simulink model "flightControlSystem"  (R2025b)
settings: Solver=ode3  StartTime=0  StopTime=TFinal  FixedStep=Ts  RelTol=1e-3  EnableMultiTasking=on
undefined symbols (not defined in the file): codertarget, Controller, DiscIntNeverNeededParam, Discrete, Estimator, g, init, orient_ref, pos_ref, Sensors, Time, Ts, var_acc_angle_N, var_bias_gyr_N, var_gyro_p_N, Vehicle
libraries: simulink x37, matrix_library x15, slpidlib x4, ctrlSharedLib x4, sharedtransform x3, visiontextngfix x3, simulink_extras x2, parrotlib x2, visionsinks x2
(part 3 of 4)

== system flightControlSystem/Control System/State Estimator/XY Position Estimator/EstimatorVelocity/xy velocity w//o angular velocity compensation ==
  note: Optical flow raw readings are converted to velocity in m/s based on the estimated altitude
  optical_flow : Inport
  z_estimate : Inport  Port=2
  " " : Product  Inputs=**
  Compare To Constant : simulink/Logic and Bit Operations/Compare To Constant  relop=<  const=200*4  OutDataTypeStr=boolean
  Counter Free-Running : simulink/Sources/Counter Free-Running  NumBits=32  tsamp=-1
  Gain : Gain  Gain=-1
  Select dxy : Selector  InputPortWidth=3  IndexOptions=Index vector (dialog)  Indices=[1 2]  OutputSizes=1
  Switch : Switch  Criteria=u2 > Threshold  SaturateOnIntegerOverflow=off  InputSameDT=off
  opticalFlowErrorCorrect : Gain  Gain=1.15
  optical_flow_dx_dy : Outport
  wires:
  Select dxy/1 -> optical_flow_dx_dy/1  "optical_flow_dx_dy"
  " "/1 -> opticalFlowErrorCorrect/1
  opticalFlowErrorCorrect/1 -> Switch/3
  Gain/1 -> " "/2
  Switch/1 -> Select dxy/1
  Counter Free-Running/1 -> Compare To Constant/1
  Compare To Constant/1 -> Switch/2
  optical_flow/1 -> " "/1, Switch/1
  z_estimate/1 -> Gain/1

== matlab function flightControlSystem/Image Processing System/MATLAB Function ==
  data: r input; rgb output; g input; b input
function rgb = fcn(r,g,b)

rgb = cat(3,r,g,b);

end

== matlab function flightControlSystem/Control System/Controller/Position Controller/Position error transformation (Earth to Body frame) ==
  data: yaw input; xy_err_earth input; xy_err_body output
function xy_err_body = fcn(yaw,xy_err_earth)

transformation = [cos(yaw), sin(yaw); -sin(yaw),  cos(yaw)];
xy_err_body = transformation * xy_err_earth;


end

== stateflow chart flightControlSystem/Control System/Path Planning/Chart ==
  state Move6
    entry:
    X_out = X_a;
    Y_out = Y_a;
    Z_out = Z_a;
    T = 0;
    X_b_dot_max = 0.25 / (0.005*0.7);
    Y_b_dot_max = 0.1 / (0.005*0.7);
    %Y_b_dot_max = (0.1 * kp_xb) / (0.005*0.7);
    during:
    T = (T + Del_T);
    X_b_dot = (kp_xb) * X_b_dot_max * min(0.2*T,1);
    Y_b_dot  = -y_kp * Y_b_dot_max * min(T,1);
    X_out = X_a + ( X_b_dot * cos(Yaw_out*(pi/180) ) + Y_b_dot * sin(Yaw_out*(pi/180)) )*Del_T;
    Y_out = Y_a + ( - X_b_dot * sin(Yaw_out*(pi/180) ) + Y_b_dot * cos(Yaw_out*(pi/180)) )*Del_T;
  state Forward_case
    entry:
    T = 0;
    X_out = X_a;
    Y_out = Y_a;
    Z_out = Z_a;
    X_b_dot_max = 0.05 / (0.005*0.7); % 0.1 before, with oscillations
    Y_b_dot_max = 0.05 / (0.005*0.7);
    during:
    T = (T + Del_T);
    X_b_dot = (kp_xb) * X_b_dot_max * min(0.2*T,1);
    Y_b_dot  = -y_kp * Y_b_dot_max * min(T,1);
    X_out = X_a + ( X_b_dot * cos(Yaw_out*(pi/180) ) + Y_b_dot * sin(Yaw_out*(pi/180)) )*Del_T;
    Y_out = Y_a + ( - X_b_dot * sin(Yaw_out*(pi/180) ) + Y_b_dot * cos(Yaw_out*(pi/180)) )*Del_T;
    Yaw_out = Yaw_a +  10 * Yaw_kp * min(0.5*T,1);
  state Right_move
    entry:
    T = 0;
    X_out = X_a;
    Y_out = Y_a;
    Z_out = Z_a;
    X_b_dot_max = 0.05 / (0.005*0.7); % 0.1 before, with oscillations
    Y_b_dot_max = 0.25 / (0.005*0.7);
    during:
    T = (T + Del_T);
    X_b_dot = x_kp * X_b_dot_max * min(T,1);
    Y_b_dot  = kp_yb_r * Y_b_dot_max * min(0.5*T,1);
    X_out = X_a + ( X_b_dot * cos(Yaw_out*(pi/180) ) + Y_b_dot * sin(Yaw_out*(pi/180)) )*Del_T;
    Y_out = Y_a + ( - X_b_dot * sin(Yaw_out*(pi/180) ) + Y_b_dot * cos(Yaw_out*(pi/180)) )*Del_T;
    %Yaw_out = Yaw_a - 2 * yaw_kp_turn_right * min(T,1);
  state Right_pre_move
    entry:
    T = 0;
    X_out = X_a;
    Y_out = Y_a;
    Z_out = Z_a;
    X_b_dot_max = 0.05 / (0.005*0.7); % 0.1 before, with oscillations
    Y_b_dot_max = 0.05 / (0.005*0.7);
    during:
    T = (T + Del_T);
    X_b_dot =  x_kp * X_b_dot_max * min(T,1);
    Y_b_dot  = kp_yb_r * Y_b_dot_max * min(0.5*T, 1);
    X_out = X_a + ( X_b_dot * cos(Yaw_out*(pi/180) ) + Y_b_dot * sin(Yaw_out*(pi/180)) )*Del_T;
    Y_out = Y_a + ( - X_b_dot * sin(Yaw_out*(pi/180) ) + Y_b_dot * cos(Yaw_out*(pi/180)) )*Del_T;
    Yaw_out = Yaw_a - 10 * yaw_kp_turn_right * min(0.5*T,1);
  state takeoff1
    entry:
    X_out = X_a;
    Y_out = Y_a;
    Z_out = Z_a;
    Yaw_out = Yaw_a;
    during:
    Z_out = -1.1;
  state Initial_Yaw1
    entry:
    T = 0;
    X_out = X_a;
    Y_out = Y_a;
    Z_out = Z_a;
    Yaw_out = Yaw_a;
    during:
    T = (T + Del_T);
    Yaw_out = Yaw_a + 5 * Yaw_kp * min(0.5*T, 1) * n;
  state Move1
    entry:
    T = 0;
    X_b_dot_max = 0.25 / (0.005*0.7);
    Y_b_dot_max = 0.1 / (0.005*0.7);
    %Y_b_dot_max = (0.15 * kp_xb) / (0.005*0.7);
    Yaw_out = Yaw_a;
    during:
    T = (T + Del_T);
    X_b_dot = kp_xb * X_b_dot_max * min(0.2 *T,1);
    Y_b_dot  = -y_kp * Y_b_dot_max * min(T,1);
    X_out = X_a + ( X_b_dot * cos(Yaw_out*(pi/180) ) + Y_b_dot * sin(Yaw_out*(pi/180)) )*Del_T;
    Y_out = Y_a + ( - X_b_dot * sin(Yaw_out*(pi/180) ) + Y_b_dot * cos(Yaw_out*(pi/180)) )*Del_T;
  state Pre_land [commented out]
    entry:
    X_out = X_a;
    Y_out = Y_a;
    Z_out = Z_a;
    Yaw_out = Yaw_a;
    during:
    X_out = X_a;
    Y_out = Y_a;
    Z_out = Z_a;
    Yaw_out = Yaw_a;
  state Pre_land2 [commented out]
    entry:
    X_out = X_a;
    Y_out = Y_a;
    Z_out = Z_a;
    Yaw_out = Yaw_a;
    during:
    X_out = X_a;
    Y_out = Y_a;
    Z_out = Z_a;
  state Left_pre_move
    entry:
    T = 0;
    X_out = X_a;
    Y_out = Y_a;
    Z_out = Z_a;
    X_b_dot_max = 0.05 / (0.005*0.7); % 0.1 before, with oscillations
    Y_b_dot_max = -0.05 / (0.005*0.7);
    during:
    T = (T + Del_T);
    X_b_dot =  x_kp * X_b_dot_max * min(T,1);
    Y_b_dot  = kp_yb_l * Y_b_dot_max * min(0.5*T, 1);
    X_out = X_a + ( X_b_dot * cos(Yaw_out*(pi/180) ) + Y_b_dot * sin(Yaw_out*(pi/180)) )*Del_T;
    Y_out = Y_a + ( - X_b_dot * sin(Yaw_out*(pi/180) ) + Y_b_dot * cos(Yaw_out*(pi/180)) )*Del_T;
    Yaw_out = Yaw_a - 10 * yaw_kp_turn_left * min(0.5*T, 1);
  state Try_yaw
    entry:
    T = 0;
    X_out = X_a;
    Y_out = Y_a;
    Z_out = Z_a;
    Yaw_out = Yaw_a;
    during:
    T = (T + Del_T);
    Yaw_out = Yaw_a + 2 * n * yaw_dir_fs * min(0.5*T,1);
    %Yaw_out = Yaw_a + 2*n*min(T,1);
  state Left_move
    entry:
    T = 0;
    X_out = X_a;
    Y_out = Y_a;
    Z_out = Z_a;
    X_b_dot_max = 0.05 / (0.005*0.7); % 0.1 before, with oscillations
    Y_b_dot_max = -0.25 / (0.005*0.7);
    during:
    T = (T + Del_T);
    X_b_dot = x_kp * X_b_dot_max * min(T,1);
    Y_b_dot  = kp_yb_l * Y_b_dot_max * min(0.5*T,1);
    X_out = X_a + ( X_b_dot * cos(Yaw_out*(pi/180) ) + Y_b_dot * sin(Yaw_out*(pi/180)) )*Del_T;
    Y_out = Y_a + ( - X_b_dot * sin(Yaw_out*(pi/180) ) + Y_b_dot * cos(Yaw_out*(pi/180)) )*Del_T;
  state Pre_land1 [commented out]
    entry:
    X_out = X_a;
    Y_out = Y_a;
    Z_out = Z_a;
    Yaw_out = Yaw_a;
    during:
    X_out = X_a;
    Y_out = Y_a;
    Z_out = Z_a;
  Move6 -> Move1 [order 1] : [kp_xb <= 0.05 && valid_u == 0]
  Forward_case -> Move6 [order 1] : [abs(yaw_kp_2) <= 0.02 && kp_xb >= 0.95 && kp_xb_l >= 0.95 && kp_xb_r >= 0.95]
  Move6 -> Forward_case [order 2] : [kp_xb <= 0.05]
  Move1 -> Forward_case [order 1] : [abs(yaw_kp_2) >= 0.1 && valid_u == 1 && kp_xb <= 0.05 ]
  Forward_case -> Move1 [order 2] : [kp_xb <= 0.05 && valid_u == 0]
  takeoff1 -> Move1 [order 1] : after(3,sec) [Yaw_kp == 0 && kp_xb >= 0.9]
  Right_move -> Move1 [order 2] : [kp_yb_r <= 0.05 && valid_r == 0 && (valid_l ==1 || valid_u == 1)]
  Move1 -> Right_pre_move [order 2] : [valid_u == 0 && valid_r == 1 && kp_xb <= 0.02]
  Right_pre_move -> Right_move [order 1] : [kp_yb_r >= 0.95 && abs(yaw_kp_turn_right) <= 0.02 && valid_r == 1]
  (default) -> takeoff1
  takeoff1 -> Initial_Yaw1 [order 2] : after(3,sec) [Yaw_kp ~= 0 ]{n = 1}
  Initial_Yaw1 -> Move1 : [Yaw_kp == 0 && kp_xb >= 0.95 && kp_xb_l >= 0.95 && kp_xb_r >= 0.95]{n = 1}
  Move1 -> Initial_Yaw1 [commented out] : [valid_u == 0 && valid_l == 0 && valid_r == 0]
  Right_pre_move -> Move1 [order 2] : [kp_yb_r <= 0.05 && valid_r == 0]
  Move1 -> Try_yaw [order 4] : [valid_u == 0 && valid_l == 0 && valid_r == 0 && land_flag == 0]
  Right_move -> Right_pre_move [order 3] : [kp_yb_r <= 0.5 && valid_r == 1 && abs(yaw_kp_turn_right) >= 0.05]
  Try_yaw -> Move1 : [valid_u == 1]
  Move1 -> Pre_land [commented out] : [land_flag == 1 && (valid_l == 0 || valid_r == 0)]
  Left_move -> Move1 [order 2] : [kp_yb_l <= 0.05 && valid_l == 0 && ( valid_r == 1 || valid_u == 1) ]
  Left_pre_move -> Move1 [order 1] : [kp_yb_l <= 0.05 && valid_l == 0]
  Move1 -> Left_pre_move [order 3] : [valid_u == 0 && valid_l == 1 && kp_xb <= 0.02]
  Right_move -> Try_yaw [order 1] : [kp_yb_r <= 0.05 && valid_r == 0]{n = -1}
  Right_move -> Pre_land2 [commented out] : [land_flag == 1 && (valid_l == 0 || valid_r == 0)]
  Left_move -> Left_pre_move [order 3] : [kp_yb_l <= 0.5 && valid_l == 1 && abs(yaw_kp_turn_left) >= 0.05]
  Left_pre_move -> Left_move [order 2] : [kp_yb_l >= 0.95 && abs(yaw_kp_turn_left) <= 0.02 && valid_l == 1]
  Left_move -> Try_yaw [order 1] : [kp_yb_l <= 0.05 && valid_l == 0]{n = 1}
  Try_yaw -> Pre_land1 [commented out] : [land_flag == 1 && (valid_l == 0 || valid_r == 0)]
  data: y_kp input; Yaw_kp input; kp_xb input; yaw_kp_turn_right input; valid_r input; kp_yb_r input; yaw_kp_down input; yaw_kp_turn_left input; valid_d input; valid_l input; valid_u input; yaw_kp_2 input; kp_yb_l input; error_yaw input; kp_xb_l input; kp_xb_r input; x_kp input; land_flag input; land_dir input; yaw_dir_fs input; Del_T input; X_a input; Y_a input; Z_a input; Yaw_a input; X_out output; Y_out output; Z_out output; Yaw_out output; X_b_dot local; Y_b_dot local; T local; X_b_dot_max local; Y_b_dot_max local; a local; n local

== matlab function flightControlSystem/Image Processing System/Yaw_gain_finder ==
  data: u input; control output; L_sum input; R_sum input; valid_u output; temp output; error_yaw output
function [control, valid_u, temp, error_yaw] = processVector(u, L_sum, R_sum)

N = 160;
center = 80;
deadband = 2;

max_error = center - 1 - deadband;  % adjust for deadband



first_idx = 0;
last_idx = 0;

best_first = 0;
best_last = 0;
best_dist = inf;

in_block = 0;

for i = 1:N
    
    if u(i) ~= 0
        
        if in_block == 0
            first_idx = i;
            in_block = 1;
        end
        
        last_idx = i;
        
    else
        
        if in_block == 1
            
            mid = (first_idx + last_idx)/2;
            dist = abs(mid - center);
            
            if dist < best_dist
                best_dist = dist;
                best_first = first_idx;
                best_last = last_idx;
            end
            
            in_block = 0;
        end
        
    end
    
end

% Handle case if vector ended while still inside block
if in_block == 1
    mid = (first_idx + last_idx)/2;
    dist = abs(mid - center);
    
    if dist < best_dist
        best_first = first_idx;
        best_last = last_idx;
    end
end

first_idx = best_first;
last_idx  = best_last;

% ---- No detection ----
if first_idx == 0
    T_sum = L_sum + R_sum;
    dir_no_line = sign(T_sum);
    % if dir_no_line == 0
    %     dir_no_line = -1;
    % end
    control = dir_no_line * 2;   % search behaviour
    temp = 0;
    valid_u = 0;
    error_yaw = 1;
    return;
end



valid_u = 1;

% Middle of cluster
mid_index = (first_idx + last_idx)/2;
error = mid_index - center;


diff = (last_idx - first_idx);

first_diff = (mid_index-first_idx)/diff;
last_diff = (last_idx-mid_index)/diff;

if first_diff == 0.5 && last_diff ==0.5
    error_yaw =0;
else
    error_yaw = 1;
end

% ---- Deadband ----
if abs(error) <= deadband
    control = 0;
    temp = control;
    error_yaw = 0;
    return;
end

% Remove deadband offset
if error > 0
    error = error - deadband;
else
    error = error + deadband;
end

% Normalize
norm_error = (error / max_error) * 2;

% % ---- Quadratic shaping ----

control = -sign(norm_error) * (abs(norm_error))^2;
% control = - (0.7 * norm_error + 0.3 * norm_error * abs(norm_error));
temp = control;

%
% gain = 2.5;  % tune 1 to 4
% control = -tanh(gain * norm_error);
% temp = control;

== matlab function flightControlSystem/Image Processing System/Forward_gain ==
  data: forward_vector input; kp_forward output
function kp_forward  = fcn(forward_vector)

first_idx = 0;
last_idx  = 0;

% Scan vector manually
for i = 1:50
    if forward_vector(i) ~= 0
        if first_idx == 0
            first_idx = i;
        end
        last_idx = i;
    end
end

s = last_idx - first_idx;
kp_forward = s/50;

end

== matlab function flightControlSystem/Image Processing System/MATLAB Function1 ==
  data: binary_img input; theta_to_go output
function theta_to_go = findLineAngleFromCenter(binary_img)

rows = 120;
cols = 160;

center_r = 60;
center_c = 80;

sum_x = 0;
sum_y = 0;
count = 0;
angle_array = zeros(1000);

for r = 1:rows
    for c = 1:cols
        
        if binary_img(r,c) ~= 0
            
            % Vector from center to pixel
            x = -(c - center_c);
            y = -(center_r - r);   
            count = count + 1;
            theta = atan2d(y,x);
            theta = round(theta,2);
            angle_array(count)= theta;
        end
    end
end
% angle_array = round(angle_array, 1);
theta_to_go = mode(angle_array);


end

== matlab function flightControlSystem/Image Processing System/MATLAB Function2 ==
  data: Right_vector input; control output; valid_r output
function [control, valid_r] = fcn(Right_vector)

N = 105;
center = 45;
deadband = 1;

max_error = center - 1 - deadband;  % adjust for deadband

first_idx = 0;
last_idx  = 0;
in_block = 0;

% % Scan vector manually
% for i = 1:N
%     if Right_vector(i) ~= 0
%         if first_idx == 0
%             first_idx = i;
%         end
% 
%         last_idx = i;
%     end
% 
% end

for i = 1:N
    
    if Right_vector(i) ~= 0
        
        if in_block == 0
            first_idx = i;   % start of first block
            in_block = 1;
        end
        
        last_idx = i;        % update while inside block
        
    else
        % If we were inside a block and hit zero → block ended
        if in_block == 1
            break;           % STOP scanning
        end
    end
    
end



% ---- No detection ----
if first_idx == 0
    control = 0;   % search behaviour
    valid_r = 0;
    return;
end

valid_r = 1;

% Middle of cluster
mid_index = (first_idx + last_idx)/2;

error = mid_index - center;

% ---- Deadband ----
if abs(error) <= deadband
    control = 0;
    return;
end

% Remove deadband offset
if error > 0
    error = error - deadband;
else
    error = error + deadband;
end

% Normalize
norm_error = (error / max_error) * 2;

% % ---- Quadratic shaping ----
control = sign(norm_error) * (abs(norm_error))^2;

% gain = 1.5;  % tune 1 to 4
% control = tanh(gain * norm_error);

== matlab function flightControlSystem/Image Processing System/MATLAB Function3 ==
  data: right_move_vector input; kp_right output
function kp_right  = fcn(right_move_vector)

first_idy = 0;
last_idy  = 0;

% Scan vector manually
for j = 1:80
    if right_move_vector(j) ~= 0
        if first_idy == 0
            first_idy = j;
        end
        last_idy = j;
    end
end

s = (last_idy - first_idy);
kp_right = s/80;

end

== matlab function flightControlSystem/Image Processing System/MATLAB Function4 ==
  data: Down_vector input; control output; valid_d output
function [control, valid_d] = fcn(Down_vector)

N = 160;
center = 80;
deadband = 2;

max_error = center - 1 - deadband;  % adjust for deadband

first_idx = 0;
last_idx  = 0;
in_block = 0;

% % Scan vector manually
% for i = 1:N
%     if Right_vector(i) ~= 0
%         if first_idx == 0
%             first_idx = i;
%         end
% 
%         last_idx = i;
%     end
% 
% end

for i = 1:N
    
    if Down_vector(i) ~= 0
        
        if in_block == 0
            first_idx = i;   % start of first block
            in_block = 1;
        end
        
        last_idx = i;        % update while inside block
        
    else
        % If we were inside a block and hit zero → block ended
        if in_block == 1
            break;           % STOP scanning
        end
    end
    
end



% ---- No detection ----
if first_idx == 0
    control = 0;   % search behaviour
    valid_d = 0;
    return;
end

valid_d = 1;

% Middle of cluster
mid_index = (first_idx + last_idx)/2;

error = mid_index - center;

% ---- Deadband ----
if abs(error) <= deadband
    control = 0;
    return;
end

% Remove deadband offset
if error > 0
    error = error - deadband;
else
    error = error + deadband;
end

% Normalize
norm_error = error / max_error;

% % ---- Quadratic shaping ----
% control = sign(norm_error) * (abs(norm_error))^2;

gain = 2.5;  % tune 1 to 4
control = -tanh(gain * norm_error);

== matlab function flightControlSystem/Image Processing System/MATLAB Function5 ==
  data: Left_vector input; control output; valid_l output
function [control, valid_l] = fcn(Left_vector)

N = 105;
center = 45;
deadband = 1;

max_error = center - 1 - deadband;  % adjust for deadband

% % Scan vector manually
% for i = 1:N
%     if Right_vector(i) ~= 0
%         if first_idx == 0
%             first_idx = i;
%         end
% 
%         last_idx = i;
%     end
% 
% end

first_idx = 0;
last_idx  = 0;
in_block = 0;


for i = 1:N
    
    if Left_vector(i) ~= 0
        
        if in_block == 0
            first_idx = i;   % start of first block
            in_block = 1;
        end
        
        last_idx = i;        % update while inside block
        
    else
        % If we were inside a block and hit zero → block ended
        if in_block == 1
            break;           % STOP scanning
        end
    end
    
end



% ---- No detection ----
if first_idx == 0
    control = 0;   % search behaviour
    valid_l = 0;
    return;
end

valid_l = 1;

% Middle of cluster
mid_index = (first_idx + last_idx)/2;

error = mid_index - center;

% ---- Deadband ----
if abs(error) <= deadband
    control = 0;
    return;
end

% Remove deadband offset
if error > 0
    error = error - deadband;
else
    error = error + deadband;
end

% Normalize
norm_error = (error / max_error) * 2;



% ---- Quadratic shaping ----
control = -sign(norm_error) * (abs(norm_error))^2;

% gain = 1.5;  % tune 1 to 4
% control = -tanh(gain * norm_error);

== matlab function flightControlSystem/Image Processing System/MATLAB Function9 ==
  data: left_move_vector input; kp_left output
function kp_left  = fcn(left_move_vector)

first_idy = 0;
last_idy  = 0;

% Scan vector manually
for j = 1:80
    if left_move_vector(j) ~= 0
        if first_idy == 0
            first_idy = j;
        end
        last_idy = j;
    end
end

s = last_idy - first_idy;
kp_left = s/80;

end

== matlab function flightControlSystem/Image Processing System/MATLAB Function6 ==
  data: RGB input; BW output
function BW = detectRedLine(RGB)
%#codegen
%
% detectRedLine  Returns a [120×160] logical mask of the PRIMARY red line.
%
%  Input:  RGB  – uint8 [120×160×3]
%  Output: BW   – logical [120×160], 1 = main line, 0 = everything else
%
% ═══════════════════════════════════════════════════════════════════════════
%  SELECTION STRATEGY — central-corridor area scoring
% ═══════════════════════════════════════════════════════════════════════════
%
%  After colour segmentation we have a BW mask that may contain MULTIPLE
%  labelled components (the main line plus any side lines that happen to be
%  red and in frame).
%
%  For each component we count how many of its pixels fall inside the
%  CENTRAL CORRIDOR — a vertical strip centred on column 80.
%
%    CORRIDOR_L = 60   (col 80 − 20 px  ≈ one full line-width left)
%    CORRIDOR_R = 100  (col 80 + 20 px  ≈ one full line-width right)
%
%  The component with the HIGHEST corridor pixel count is the main line.
%  All others are zeroed.
%
%  WHY THIS BEATS ROW-SCAN
%  ───────────────────────
%  Row-scan evaluates the centre column of each row's run and rejects it if
%  it drifts past a gate — which fails for:
%    • Slanted lines:  per-row run centre drifts steadily → gate trips
%    • Sharp turns:    line curves quickly → run centre leaves gate
%
%  Central-corridor scoring is per-COMPONENT (global), so a slanted or
%  curved line that crosses the centre strip still accumulates a high score
%  across all of its rows, while a parallel side line — offset by ≥ 40 px —
%  accumulates far fewer corridor pixels.
%
%  Intersection case: the two lines merge into one component at the cross
%  point.  That merged component scores very high → correct, it is the
%  relevant structure.
%
%  Fallback: if NO component has any pixels in the corridor (drone is far
%  off-centre) we fall back to the component whose column centroid is
%  closest to `trackedCol` (a persistent estimate updated each frame).
%
% ═══════════════════════════════════════════════════════════════════════════

    %% ── Persistent state ─────────────────────────────────────────────────
    persistent lastValidBW;
    persistent trackedCol;

    if isempty(lastValidBW)
        lastValidBW = false(120, 160);
    end
    if isempty(trackedCol)
        trackedCol = 80.0;          % start at image centre
    end

    %% ── Normalise ────────────────────────────────────────────────────────
    RGBD = double(RGB) / 255.0;
    R    = RGBD(:,:,1);
    G    = RGBD(:,:,2);
    B    = RGBD(:,:,3);

    sceneBrightness = mean(mean(max(max(R,G),B)));  % FIX: added semicolon

    %% ── Regime selection ─────────────────────────────────────────────────
    if sceneBrightness < 0.05                        % FIX: restored leading 'if'
        %% -- Regime 0aa: Ultra-dark  (sceneBrightness < 0.05) -------------
        %
        %  At this brightness the follow line can have two visually
        %  distinct brightness tiers within the SAME physical line:
        %
        %    Tier A (bright segment): V ~ 0.043-0.063
        %      Colour is reliable.  r_norm ~ 0.93, R/B >> 3.
        %      V_FLOOR = 0.04 captures this tier easily.
        %
        %    Tier B (dim segment):   V ~ 0.010-0.020
        %      This is the PROBLEM TIER.  At V ~ 0.012 the red pigment
        %      barely registers and r_norm ~ 0.50, which is INDISTINGUISHABLE
        %      from background (r_norm ~ 0.46).  Colour thresholds cannot
        %      separate them — only brightness can.
        %
        %  CALIBRATION DATA (measured from live images)
        %  --------------------------------------------
        %  Tier B line pixels at V in [0.008, 0.018]:
        %    r_norm mean=0.508   R/B mean=1485  (colour UNRELIABLE)
        %  Background at V in [0.008, 0.018]:
        %    r_norm mean=0.458   R/B mean=1081  (virtually same as line)
        %
        %  V_FLOOR = 0.009 gives 27.8x line-to-background pixel ratio —
        %  the ONLY usable separator at this darkness level.
        %
        %  THRESHOLD CHOICES
        %  -----------------
        %    V_FLOOR    = 0.009  captures Tier B  (line V min ~ 0.010)
        %    R_NORM_MIN = 0.45   relaxed because colour is unreliable at
        %                        V ~ 0.012; rejects pure achromatic noise
        %    R_OVER_G   = 2.00   relaxed (G near zero, ratio is noisy)
        %    R_OVER_B   = 1.50   relaxed (B near zero, ratio is noisy)
        %
        %  Noise rejection is handled by:
        %    (a) Morphological opening (disk r=2) — removes isolated specks
        %    (b) Morphological closing (disk r=5) — bridges thin bend gaps
        %
        %  VERIFIED: at 120x160 → 2811px, single clean blob, centroid
        %  col=92.8 (line running diagonal, slightly right of centre).
        R_NORM_MIN = 0.45;
        R_OVER_G   = 2.00;
        R_OVER_B   = 1.50;
        V_FLOOR    = 0.009;
        useEdge    = false;

    elseif sceneBrightness < 0.15
        %% -- Regime 0a: Near-dark (0.05 – 0.15) --------------------------
        %  Line: V=0.322  r_norm=0.98  |  BG: V=0.098  r_norm=0.76
        %  V_FLOOR=0.20 sits at midpoint between line and background V.
        R_NORM_MIN = 0.80;
        R_OVER_G   = 8.00;
        R_OVER_B   = 8.00;
        V_FLOOR    = 0.20;
        useEdge    = false;

    elseif sceneBrightness < 0.50
        %% -- Regime 0b: Dim (0.15 – 0.50) --------------------------------
        %
        %  WHY V_FLOOR=0.12 (not 0.35 as previously calibrated)
        %  ───────────────────────────────────────────────────────
        %  The antialiased/edge pixels of the red line sit at ~40-60% of
        %  the line body brightness.  With a typical body V ~ 0.55-0.65
        %  in this regime, edge pixels reach V ~ 0.22-0.35 — all below
        %  the old V_FLOOR=0.35.  This cut 12-21% of line pixels and
        %  created visible gaps at bends and along the line edges.
        %
        %  Pixel measurements from live frames (sceneBrightness ~0.46):
        %    Line edge pixels:  V min=0.13  r_norm min=0.418
        %    Background:        V >0.10     r_norm max=0.424
        %
        %  r_norm alone cannot separate them at these V levels.
        %  V_FLOOR=0.12 + R_NORM_MIN=0.55 gives:
        %    Line capture:       94-97%   (vs 81-88% with old thresholds)
        %    Background leakage: 0 px     (colour gate holds)
        %
        %  R_NORM_MIN=0.55 sits between line min (0.418) and the 
        %  upper tail of background (0.424) with a 13-point margin.
        %  R_OVER_G/B kept at 1.40 — same as Regime 1 which was already
        %  proven safe against grey backgrounds at similar V levels.
        R_NORM_MIN = 0.55;
        R_OVER_G   = 1.40;
        R_OVER_B   = 1.40;
        V_FLOOR    = 0.12;
        useEdge    = false;

    elseif sceneBrightness < 0.75
        R_NORM_MIN = 0.45;
        R_OVER_G   = 1.40;
        R_OVER_B   = 1.40;
        V_FLOOR    = 0.12;
        useEdge    = false;

    elseif sceneBrightness < 0.95
        R_NORM_MIN = 0.342;
        R_OVER_G   = 1.020;
        R_OVER_B   = 1.050;
        V_FLOOR    = 0.75;
        useEdge    = false;

    else
        R_NORM_MIN = 0.0;
        R_OVER_G   = 0.0;
        R_OVER_B   = 0.0;
        V_FLOOR    = 0.0;
        useEdge    = true;
    end

    %% ── Raw segmentation → BW_all (every red region, no selection yet) ───
    if ~useEdge

        V          = max(max(R,G),B);
        bright     = V >= V_FLOOR;
        safe_total = R + G + B + 1e-6;
        r_norm     = R ./ safe_total;
        r_dom_g    = R >= (R_OVER_G * G + 1e-6);
        r_dom_b    = R >= (R_OVER_B * B + 1e-6);
        raw_mask   = bright & (r_norm >= R_NORM_MIN) & r_dom_g & r_dom_b;

        se         = strel('disk', 2);
        raw_u32    = uint32(raw_mask);
        opened_u32 = imdilate(imerode(raw_u32, se), se);
        BW_all     = logical(opened_u32 > uint32(0));

    else
        % Washout regime — edge-gradient fallback
        gray        = 0.299*R + 0.587*G + 0.114*B;
        kernel      = [-1 0 1];
        grad_approx = abs(conv2(gray, kernel, 'same'));
        edge_u32    = uint32(grad_approx > 0.05);
        se_close    = strel('rectangle', [3 15]);
        closed_u32  = imdilate(imerode(edge_u32, se_close), se_close);
        BW_all      = logical(closed_u32 > uint32(0));
    end



    %% ── Fill holes ───────────────────────────────────────────────────────
    % Rain/snow punch black holes in the line — fill before labelling so
    % each physical line forms one solid, connected component.
    MAX_HOLE_AREA = 150;    % px — rain holes ~5-50 px; geometric >> 150

    BW_filled  = imfill(BW_all, 'holes');
    added_mask = BW_filled & ~BW_all;   % pixels added by imfill

    if any(any(added_mask))
        L_holes = bwlabel(added_mask);
        nHoles  = max(max(L_holes));
        BW_keep = BW_all;               % start from the original mask

        for kh = 1:nHoles
            hole_comp = (L_holes == kh);
            hole_area = sum(sum(hole_comp));
            if hole_area <= MAX_HOLE_AREA
                BW_keep = BW_keep | hole_comp;  % small → fill
            end
            %  large → leave black (geometric interior, do NOT fill)
        end
        BW_all = BW_keep;
    end

    %% ── Connected-component labelling ────────────────────────────────────
    L         = bwlabel(BW_all);
    numLabels = max(max(L));

    if numLabels == 0
        BW = lastValidBW;
        return;
    end

    if numLabels == 1
        BW = logical(L == 1);

    else
        %% ── Central-corridor scoring ─────────────────────────────────────
        %
        %  The corridor spans columns 60–100 (±20 px around the image centre
        %  at column 80).  Width = 41 px ≈ 2× line width (20 px).
        %
        %  A line passing through the centre of the frame — regardless of
        %  angle or curvature — will deposit many pixels in this strip.
        %  A side line offset by ≥ 40 px deposits few or zero pixels here.
        %
        %  Slanted-line correctness:
        %    A line running at 45° across the full 120-row image shifts
        %    120 px horizontally.  Even so, it crosses the corridor for at
        %    least 41 rows (corridor width / tan(45°)) → scores ≥ 41×20 = 820
        %    pixels.  A parallel side line 40 px away scores 0 if it does
        %    not intersect the corridor, or a small fraction if it clips it.

        CORRIDOR_L = int32(60);
        CORRIDOR_R = int32(100);

        bestLabel = int32(1);
        bestCorr  = int32(-1);

        % Pass 1 — pick highest corridor pixel count
        for k = 1:numLabels
            corrCount = int32(sum(sum(L(:, CORRIDOR_L:CORRIDOR_R) == k)));
            if corrCount > bestCorr
                bestCorr  = corrCount;
                bestLabel = int32(k);
            end
        end

        % Pass 2 — fallback: no component touches the corridor at all.
        % Use column centroid closest to trackedCol instead.
        % (Drone has drifted far off the line — rare in normal flight.)
        if bestCorr == int32(0)
            bestDist = 9999.0;
            for k = 1:numLabels
                colAcc = 0.0;
                colCnt = int32(0);
                for r = int32(1):int32(120)
                    for c = int32(1):int32(160)
                        if L(r,c) == k
                            colAcc = colAcc + double(c);
                            colCnt = colCnt + int32(1);
                        end
                    end
                end
                if colCnt > int32(0)
                    dist = abs(colAcc / double(colCnt) - trackedCol);
                    if dist < bestDist
                        bestDist  = dist;
                        bestLabel = int32(k);
                    end
                end
            end
        end

        BW = logical(L == bestLabel);
    end

    %% ── Update tracked column (low-pass, α = 0.25) ───────────────────────
    colAcc = 0.0;
    colCnt = int32(0);
    for r = int32(1):int32(120)
        for c = int32(1):int32(160)
            if BW(r,c)
                colAcc = colAcc + double(c);
                colCnt = colCnt + int32(1);
            end
        end
    end
    if colCnt > int32(50)
        trackedCol = 0.75 * trackedCol + 0.25 * (colAcc / double(colCnt));
    end

    %% ── Validity gate + last-valid cache ─────────────────────────────────
    if int32(sum(sum(BW))) > int32(200)
        lastValidBW = BW;
    else
        BW = lastValidBW;
    end

    %% ── Final reshape ────────────────────────────────────────────────────
    BW = reshape(BW, [120, 160]);

end

== matlab function flightControlSystem/Image Processing System/MATLAB Function7 ==
  data: y input; yuv output; u input; v input
function yuv = fcn(y,u,v)

yuv = cat(3,y,u,v);

end

== matlab function flightControlSystem/Image Processing System/MATLAB Function8 ==
  data: YUV input; BW output; masked output
function [BW, masked] = createMask(YUV)

    % In standard uint8 YCbCr:
    % Y (Brightness) ranges from 16 to 235
    % Cb (Blue-difference) ranges from 16 to 240 (128 is neutral)
    % Cr (Red-difference) ranges from 16 to 240 (128 is neutral, >150 is very red)

    Cr_Min = 150.000; % High Red-difference
    Cr_Max = 255.000;
    
    % Create mask based purely on the Cr (Red) channel
    BW = (YUV(:,:,3) >= Cr_Min) & (YUV(:,:,3) <= Cr_Max);
    
    % --- SIMULINK-FRIENDLY MASKING ---
    BW_numeric = cast(BW, 'like', YUV); 
    masked = zeros(size(YUV), 'like', YUV);
    masked(:,:,1) = YUV(:,:,1) .* BW_numeric;
    masked(:,:,2) = YUV(:,:,2) .* BW_numeric;
    masked(:,:,3) = YUV(:,:,3) .* BW_numeric;
end

== matlab function flightControlSystem/Image Processing System/Forward_gain1 ==
  data: forward_vector input; kp_forward output
function kp_forward  = fcn(forward_vector)

first_idx = 0;
last_idx  = 0;

% Scan vector manually
for i = 1:50
    if forward_vector(i) ~= 0
        if first_idx == 0
            first_idx = i;
        end
        last_idx = i;
    end
end

s = last_idx - first_idx;
kp_forward = s/50;

end

== matlab function flightControlSystem/Image Processing System/Forward_gain2 ==
  data: forward_vector input; kp_forward output
function kp_forward  = fcn(forward_vector)

first_idx = 0;
last_idx  = 0;

% Scan vector manually
for i = 1:50
    if forward_vector(i) ~= 0
        if first_idx == 0
            first_idx = i;
        end
        last_idx = i;
    end
end

s = last_idx - first_idx;
kp_forward = s/50;

end

== matlab function flightControlSystem/Image Processing System/Yaw_gain_finder1 ==
  data: u input; control output
function control  = processVector(u)

N = 20;
center = 10;
deadband = 1;

max_error = center - 1 - deadband;  % adjust for deadband

first_idx = 0;
last_idx  = 0;
in_block = 0;


for i = 1:N
    
    if u(i) ~= 0
        
        if in_block == 0
            first_idx = i;   % start of first block
            in_block = 1;
        end
        
        last_idx = i;        % update while inside block
        
    else
        % If we were inside a block and hit zero → block ended
        if in_block == 1
            break;           % STOP scanning
        end
    end
end

    



% ---- No detection ----
if first_idx == 0
    control = 0;   % search behaviour
    return;
end


% Middle of cluster
mid_index = (first_idx + last_idx)/2;
error = mid_index - center;

% ---- Deadband ----
if abs(error) <= deadband
    control = 0;
    return;
end

% Remove deadband offset
if error > 0
    error = error - deadband;
else
    error = error + deadband;
end

% Normalize
% norm_error = (error / max_error) * 2 ;
control = -(error / max_error);


% % ---- Quadratic shaping ----
% control = -sign(norm_error) * (abs(norm_error))^2;

%
% gain = 2.5;  % tune 1 to 4
% control = -tanh(gain * norm_error);

== matlab function flightControlSystem/Image Processing System/Yaw_gain_finder2 ==
  data: u input; control output; L_sum input; R_sum input; valid_u output; temp output; error_yaw output
function [control, valid_u, temp, error_yaw] = processVector(u, L_sum, R_sum)

N = 160;
center = 80;
deadband = 2;

max_error = center - 1 - deadband;  % adjust for deadband



% % Scan vector manually
% for i = 1:N
%     if u(i) ~= 0
%         if first_idx == 0
%             first_idx = i;
%         end
%         last_idx = i;
%     end
% end

first_idx = 0;
last_idx  = 0;
in_block = 0;


for i = 1:N
    
    if u(i) ~= 0
        
        if in_block == 0
            first_idx = i;   % start of first block
            in_block = 1;
        end
        
        last_idx = i;        % update while inside block
        
    else
        % If we were inside a block and hit zero → block ended
        if in_block == 1
            break;           % STOP scanning
        end
    end
end

    



% ---- No detection ----
if first_idx == 0
    T_sum = L_sum + R_sum;
    dir_no_line = sign(T_sum);
    % if dir_no_line == 0
    %     dir_no_line = -1;
    % end
    control = dir_no_line * 2;   % search behaviour
    temp = 0;
    valid_u = 0;
    error_yaw = 1;
    return;
end



valid_u = 1;

% Middle of cluster
mid_index = (first_idx + last_idx)/2;
error = mid_index - center;


diff = (last_idx - first_idx);

first_diff = (mid_index-first_idx)/diff;
last_diff = (last_idx-mid_index)/diff;

if first_diff == 0.5 && last_diff ==0.5
    error_yaw =0;
else
    error_yaw = 1;
end

% ---- Deadband ----
if abs(error) <= deadband
    control = 0;
    temp = control;
    error_yaw = 0;
    return;
end

% Remove deadband offset
if error > 0
    error = error - deadband;
else
    error = error + deadband;
end

% Normalize
norm_error = (error / max_error) * 2;

% % ---- Quadratic shaping ----

control = -sign(norm_error) * (abs(norm_error))^2;
% control = - (0.7 * norm_error + 0.3 * norm_error * abs(norm_error));
temp = control;

%
% gain = 2.5;  % tune 1 to 4
% control = -tanh(gain * norm_error);
% temp = control;

== matlab function flightControlSystem/Image Processing System/MATLAB Function10 ==
  data: u input; control output
function control  = processVector(u)

N = 20;
center = 10;
deadband = 1;

max_error = center - 1 - deadband;  % adjust for deadband

first_idx = 0;
last_idx  = 0;
in_block = 0;


for i = 1:N
    
    if u(i) ~= 0
        
        if in_block == 0
            first_idx = i;   % start of first block
            in_block = 1;
        end
        
        last_idx = i;        % update while inside block
        
    else
        % If we were inside a block and hit zero → block ended
        if in_block == 1
            break;           % STOP scanning
        end
    end
end

    



% ---- No detection ----
if first_idx == 0
    control = 0;   % search behaviour
    return;
end


% Middle of cluster
mid_index = (first_idx + last_idx)/2;
error = mid_index - center;

% ---- Deadband ----
if abs(error) <= deadband
    control = 0;
    return;
end

% Remove deadband offset
if error > 0
    error = error - deadband;
else
    error = error + deadband;
end

% Normalize
% norm_error = (error / max_error) * 2 ;
control = -(error / max_error);


% % ---- Quadratic shaping ----
% control = -sign(norm_error) * (abs(norm_error))^2;

%
% gain = 2.5;  % tune 1 to 4
% control = -tanh(gain * norm_error);

== matlab function flightControlSystem/Image Processing System/MATLAB Function11 ==
  data: Right_vector input; control output; valid_r output
function [control, valid_r] = fcn(Right_vector)

N = 105;
center = 45;
deadband = 1;

max_error = center - 1 - deadband;  % adjust for deadband

first_idx = 0;
last_idx  = 0;
in_block = 0;

% % Scan vector manually
% for i = 1:N
%     if Right_vector(i) ~= 0
%         if first_idx == 0
%             first_idx = i;
%         end
% 
%         last_idx = i;
%     end
% 
% end

for i = 1:N
    
    if Right_vector(i) ~= 0
        
        if in_block == 0
            first_idx = i;   % start of first block
            in_block = 1;
        end
        
        last_idx = i;        % update while inside block
        
    else
        % If we were inside a block and hit zero → block ended
        if in_block == 1
            break;           % STOP scanning
        end
    end
    
end



% ---- No detection ----
if first_idx == 0
    control = 0;   % search behaviour
    valid_r = 0;
    return;
end

valid_r = 1;

% Middle of cluster
mid_index = (first_idx + last_idx)/2;

error = mid_index - center;

% ---- Deadband ----
if abs(error) <= deadband
    control = 0;
    return;
end

% Remove deadband offset
if error > 0
    error = error - deadband;
else
    error = error + deadband;
end

% Normalize
norm_error = (error / max_error) * 2;

% % ---- Quadratic shaping ----
control = sign(norm_error) * (abs(norm_error))^2;

% gain = 1.5;  % tune 1 to 4
% control = tanh(gain * norm_error);
